simulink model "TestHeightController"  (R2020b)
settings: Solver=VariableStepAuto  StartTime=0.0  StopTime=10.0  RelTol=1e-3
undefined symbols (not defined in the file): Initial, Uav
libraries: pid_lib x1
settings Model: Creator=jban039  LastModifiedBy=jeremie
settings DebuggingCC: ArithmeticOperatorsInVariantConditions=warning
settings SFSimCC: SimUseLocalCustomCode=off  CustomCodeUndefinedFunction=UseInterfaceOnly
settings RTWCC: RTWUseLocalCustomCode=off

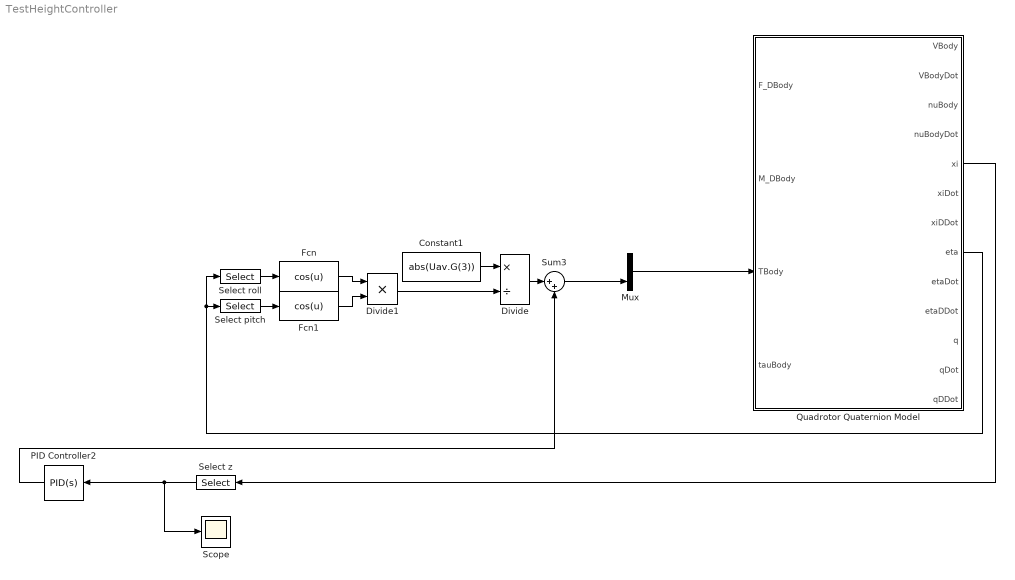
== system TestHeightController ==
  Constant1 : Constant  Value=abs(Uav.G(3))
  Divide : Product  Inputs=*/
  Divide1 : Product  Inputs=**
  Fcn : Fcn  Expr=cos(u)
  Fcn1 : Fcn  Expr=cos(u)
  Mux : Mux  Inputs=3
  PID Controller2 : pid_lib/PID Controller  Controller=PID  Form=Parallel  TimeDomain=Continuous-time  UseExternalTs=off  SampleTime=-1  IntegratorMethod=Forward Euler  FilterMethod=Forward Euler  ControllerParametersSource=internal  P=-22.065410118279  I=-10.2297340963903  D=-11.7817329577601  UseFilter=on  N=104.897155810233  TunerSelectOption=Transfer Function Based (PID Tuner App)  InitialConditionSource=internal  InitialConditionForIntegrator=0  InitialConditionForFilter=0  DifferentiatorICPrevScaledInput=0  ExternalReset=none  TrackingMode=off  Kt=1  LimitOutput=off  SatLimitsSource=internal  UpperSaturationLimit=inf  LowerSaturationLimit=-inf  LinearizeAsGain=on  AntiWindupMode=none  Kb=1  POutMin=[]  POutMax=[]  IOutMin=[]  IOutMax=[]  DOutMin=[]  DOutMax=[]  NOutMin=[]  NOutMax=[]  SumOutMin=[]  SumOutMax=[]  SaturationOutMin=[]  SaturationOutMax=[]  PParamMin=[]  PParamMax=[]  IParamMin=[]  IParamMax=[]  DParamMin=[]  DParamMax=[]  NParamMin=[]  NParamMax=[]  KbParamMin=[]  KbParamMax=[]  KtParamMin=[]  KtParamMax=[]  KbOutMin=[]  KbOutMax=[]  KtOutMin=[]  KtOutMax=[]  IntegratorOutMin=[]  IntegratorOutMax=[]  FilterOutMin=[]  FilterOutMax=[]  SumI1OutMin=[]  SumI1OutMax=[]  SumI2OutMin=[]  SumI2OutMax=[]  SumI3OutMin=[]  SumI3OutMax=[]  SumI4OutMin=[]  SumI4OutMax=[]  SumDOutMin=[]  SumDOutMax=[]  DifferentiatorOutMin=[]  DifferentiatorOutMax=[]  FilterDiffOutCoefMin=[]  FilterDiffOutCoefMax=[]  ReciprocalOutMin=[]  ReciprocalOutMax=[]  SumDenOutMin=[]  SumDenOutMax=[]  SumNumOutMin=[]  SumNumOutMax=[]  DivideOutMin=[]  DivideOutMax=[]  UdiffTsProdOutMin=[]  UdiffTsProdOutMax=[]  NTsProdOutMin=[]  NTsProdOutMax=[]  UintegralTsProdOutMin=[]  UintegralTsProdOutMax=[]  UngainTsProdOutMin=[]  UngainTsProdOutMax=[]  IntegratorContinuousStateAttributes=''  IntegratorStateMustResolveToSignalObject=off  IntegratorRTWStateStorageClass=Auto  FilterContinuousStateAttributes=''  FilterStateMustResolveToSignalObject=off  FilterRTWStateStorageClass=Auto  ParallelPVariant=InternalParameters  IdealPVariant=Disabled  IVariant=InternalParameters  DVariant=InternalParameters  IntegratorVariant=Continuous  SatVariant=Disabled  AWVariant=Passthrough  PCopyVariant=Disabled  TRVariant=Disabled  FdbkBlocksVariant=Forward  IdealPFdbkVariant=Disabled  SatFdbkVariant=Disabled  DerivativeFilterVariant=ContFilter  NVariant=InternalParameters  NCopyVariant=Disabled  FilterICVariant=InternalICsFilter  IntegratorICVariant=InternalICs  ExternalResetVariant=Disabled  TRSumVariant=Passthrough  SumFdbkVariant=Disabled  SumVariant=Sum_PID  TsampFilterVariant=InternalTs  TsampNgainVariant=Passthrough  TsampIntegralVariant=Passthrough  ExternalSaturationOutDataTypeStr=Inherit: Same as second input
  Quadrotor Quaternion Model : Subsystem
  Scope : Scope
  Select pitch : Selector  InputPortWidth=3  IndexOptions=Index vector (dialog)  Indices=2  OutputSizes=1
  Select roll : Selector  InputPortWidth=3  IndexOptions=Index vector (dialog)  Indices=1  OutputSizes=1
  Select z : Selector  InputPortWidth=3  IndexOptions=Index vector (dialog)  Indices=3  OutputSizes=1
  Sum3 : Sum  Inputs=|++
  wires:
  PID Controller2/1 -> Sum3/2
  Divide1/1 -> Divide/2
  Fcn1/1 -> Divide1/2
  Fcn/1 -> Divide1/1
  Select pitch/1 -> Fcn1/1
  Select roll/1 -> Fcn/1
  Quadrotor Quaternion Model/8(eta) -> Select pitch/1, Select roll/1
  Constant1/1 -> Divide/1
  Divide/1 -> Sum3/1
  Sum3/1 -> Mux/3
  Mux/1 -> Quadrotor Quaternion Model/3(TBody)
  Quadrotor Quaternion Model/5(xi) -> Select z/1
  Select z/1 -> Scope/1, PID Controller2/1

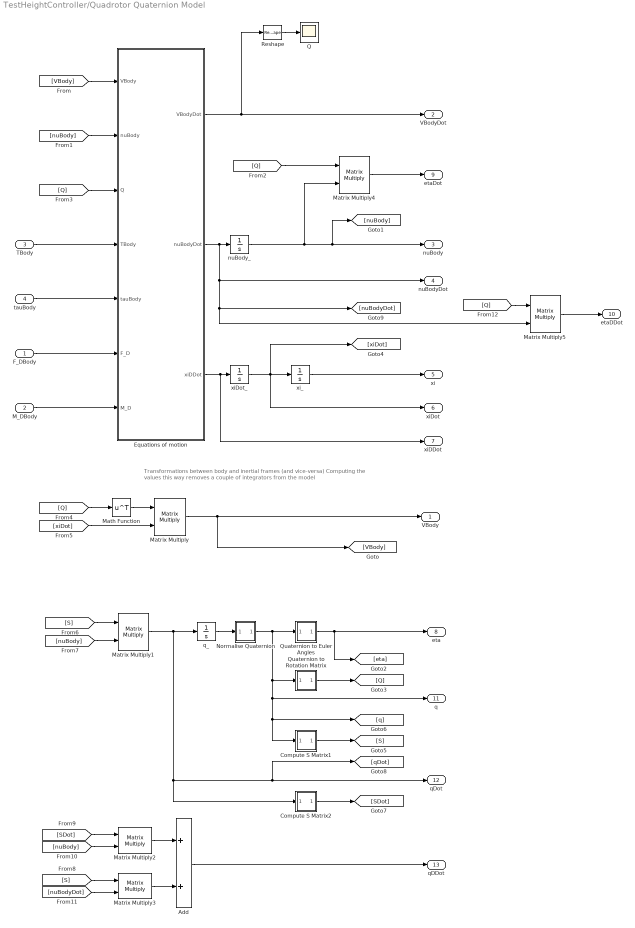
== system TestHeightController/Quadrotor Quaternion Model ==
  note: Transformations between body and inertial frames (and vice-versa)
      | Computing the values this way removes a couple of integrators from the model
  F_DBody : Inport  Unit=N
  M_DBody : Inport  Port=2  Unit=N*m
  TBody : Inport  Port=3  Unit=N
  tauBody : Inport  Port=4  Unit=N*m
  Add : Sum
  Compute S Matrix1 : Subsystem  AncestorBlock=QuaternionLibrary/Compute S Matrix
      mask help: Convert an orientation quaternion to an orthogonal transformation matrix
      mask Help:
      | Convert a quaternion
      | [q1 q2 q3 q4]
      | to the S matrix used to compute angular acceleration and velocity quaternion
      | qDot = S * nuBody
      | 
      | qDDot = SDot * nuBody + S * nuBodyDot
      mask Display: disp('S')
  Compute S Matrix2 : Subsystem  AncestorBlock=QuaternionLibrary/Compute S Matrix
      mask help: Convert an orientation quaternion to an orthogonal transformation matrix
      mask Help:
      | Convert a quaternion
      | [q1 q2 q3 q4]
      | to the S matrix used to compute angular acceleration and velocity quaternion
      | qDot = S * nuBody
      | 
      | qDDot = SDot * nuBody + S * nuBodyDot
      mask Display: disp('S')
  Equations of motion : MATLAB Function  TreatAsAtomicUnit=on
  Math Function : Math  Operator=transpose  SignedPower=on  SaturateOnIntegerOverflow=on
  Matrix Multiply{,1..5} (6 alike) : Product  Multiplication=Matrix(*)
  Normalise Quaternion : Subsystem  AncestorBlock=QuaternionLibrary/Normalise Quaternion
      mask help:
      | Normalise a quaternion
      |
      | Qhat = Q / |Q|
      mask Display: disp('Q/|Q|')
  Q : Scope
  Quaternion to Euler Angles : Subsystem  AncestorBlock=QuaternionLibrary/Quaternion to Euler Angles
      mask help: Convert an orientation quaternion to a vector of Euler angles
      mask Help:
      | Convert an orientation quaternion
      | [q1 q2 q3 q4]
      | where:
      | - q1 is the rotation in radians
      | - [q2 q3 q4] is the vector around which the rotation is performed)
      | to a vector of Euler angles
      | [roll, pitch, yaw]
      | Based on code from the PX4 firmware: https://github.com/PX4/Firmware
      mask Display: disp('Q2E')
  Quaternion to Rotation Matrix : Subsystem  AncestorBlock=QuaternionLibrary/Quaternion to Rotation Matrix
      mask help: Convert an orientation quaternion to an orthogonal transformation matrix
      mask Help:
      | Convert an orientation quaternion
      | [q1 q2 q3 q4]
      | where:
      | - q1 is the rotation in radians
      | - [q2 q3 q4] is the vector around which the rotation is performed)
      | to an orthogonal transformation matrix
      | Based on code from the PX4 firmware: https://github.com/PX4/Firmware
      mask Display: disp('Q2R')
  Reshape : Reshape  OutputDimensionality=Column vector (2-D)
  nuBody_ : Integrator  InitialCondition=Initial.NU_BODY
  q_ : Integrator  InitialCondition=Initial.Q
  xiDot_ : Integrator  InitialCondition=Initial.XI_DOT
  xi_ : Integrator  InitialCondition=[0;0;0.01]
  VBody : Outport  Unit=m/s  VectorParamsAs1DForOutWhenUnconnected=off
  VBodyDot : Outport  Port=2  Unit=m/s^2  VectorParamsAs1DForOutWhenUnconnected=off
  nuBody : Outport  Port=3  Unit=rad/s  VectorParamsAs1DForOutWhenUnconnected=off
  nuBodyDot : Outport  Port=4  Unit=rad/s^2  VectorParamsAs1DForOutWhenUnconnected=off
  xi : Outport  Port=5  Unit=m  VectorParamsAs1DForOutWhenUnconnected=off
  xiDot : Outport  Port=6  Unit=m/s  VectorParamsAs1DForOutWhenUnconnected=off
  xiDDot : Outport  Port=7  Unit=m/s^2  VectorParamsAs1DForOutWhenUnconnected=off
  eta : Outport  Port=8  Unit=rad  VectorParamsAs1DForOutWhenUnconnected=off
  etaDot : Outport  Port=9  Unit=rad/s  VectorParamsAs1DForOutWhenUnconnected=off
  etaDDot : Outport  Port=10  Unit=rad/s^2  VectorParamsAs1DForOutWhenUnconnected=off
  q : Outport  Port=11  VectorParamsAs1DForOutWhenUnconnected=off
  qDot : Outport  Port=12  VectorParamsAs1DForOutWhenUnconnected=off
  qDDot : Outport  Port=13  VectorParamsAs1DForOutWhenUnconnected=off
  wires:
  xiDot_/1 -> xiDot/1, [xiDot], xi_/1
  Reshape/1 -> Q/1
  Matrix Multiply5/1 -> etaDDot/1
  [Q] -> Matrix Multiply5/1
  Add/1 -> qDDot/1
  [Q] -> Matrix Multiply4/1
  Compute S Matrix1/1(rotationMatrix) -> [S]
  Normalise Quaternion/1(normalised) -> Quaternion to Rotation Matrix/1(quaternion), [q], Compute S Matrix1/1(quaternion), q/1, Quaternion to Euler Angles/1(quaternion)
  Matrix Multiply3/1 -> Add/2
  Matrix Multiply2/1 -> Add/1
  [nuBodyDot] -> Matrix Multiply3/2
  [nuBody] -> Matrix Multiply2/2
  [SDot] -> Matrix Multiply2/1
  Matrix Multiply1/1 -> q_/1, Compute S Matrix2/1(quaternion), [qDot], qDot/1
  [S] -> Matrix Multiply3/1
  Compute S Matrix2/1(rotationMatrix) -> [SDot]
  [nuBody] -> Matrix Multiply1/2
  [S] -> Matrix Multiply1/1
  Math Function/1 -> Matrix Multiply/1
  [xiDot] -> Matrix Multiply/2
  [Q] -> Math Function/1
  [Q] -> Equations of motion/3(Q)
  Quaternion to Rotation Matrix/1(rotationMatrix) -> [Q]
  Matrix Multiply4/1 -> etaDot/1
  Quaternion to Euler Angles/1(euler) -> [eta], eta/1
  q_/1 -> Normalise Quaternion/1(quaternion)
  Equations of motion/2(nuBodyDot) -> [nuBodyDot], Matrix Multiply5/2, nuBodyDot/1, nuBody_/1
  nuBody_/1 -> nuBody/1, [nuBody], Matrix Multiply4/2
  M_DBody/1 -> Equations of motion/7(M_D)
  Matrix Multiply/1 -> [VBody], VBody/1
  F_DBody/1 -> Equations of motion/6(F_D)
  Equations of motion/3(xiDDot) -> xiDDot/1, xiDot_/1
  TBody/1 -> Equations of motion/4(TBody)
  tauBody/1 -> Equations of motion/5(tauBody)
  [VBody] -> Equations of motion/1(VBody)
  [nuBody] -> Equations of motion/2(nuBody)
  xi_/1 -> xi/1
  Equations of motion/1(VBodyDot) -> VBodyDot/1, Reshape/1

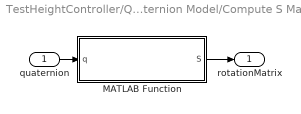
== system TestHeightController/Quadrotor Quaternion Model/Compute S Matrix1 ==
  quaternion : Inport
  MATLAB Function : MATLAB Function  TreatAsAtomicUnit=on
  rotationMatrix : Outport  VectorParamsAs1DForOutWhenUnconnected=off
  wires:
  quaternion/1 -> MATLAB Function/1(q)
  MATLAB Function/1(S) -> rotationMatrix/1

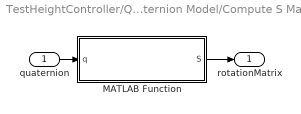
== system TestHeightController/Quadrotor Quaternion Model/Compute S Matrix2 ==
  quaternion : Inport
  MATLAB Function : MATLAB Function  TreatAsAtomicUnit=on
  rotationMatrix : Outport  VectorParamsAs1DForOutWhenUnconnected=off
  wires:
  quaternion/1 -> MATLAB Function/1(q)
  MATLAB Function/1(S) -> rotationMatrix/1

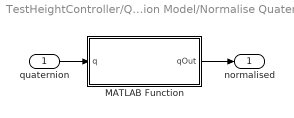
== system TestHeightController/Quadrotor Quaternion Model/Normalise Quaternion ==
  quaternion : Inport
  MATLAB Function : MATLAB Function  TreatAsAtomicUnit=on
  normalised : Outport  VectorParamsAs1DForOutWhenUnconnected=off
  wires:
  quaternion/1 -> MATLAB Function/1(q)
  MATLAB Function/1(qOut) -> normalised/1

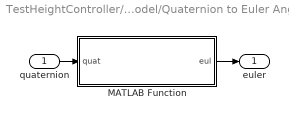
== system TestHeightController/Quadrotor Quaternion Model/Quaternion to Euler Angles ==
  quaternion : Inport
  MATLAB Function : MATLAB Function  TreatAsAtomicUnit=on
  euler : Outport  VectorParamsAs1DForOutWhenUnconnected=off
  wires:
  quaternion/1 -> MATLAB Function/1(quat)
  MATLAB Function/1(eul) -> euler/1

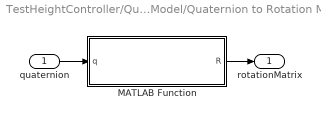
== system TestHeightController/Quadrotor Quaternion Model/Quaternion to Rotation Matrix ==
  quaternion : Inport
  MATLAB Function : MATLAB Function  TreatAsAtomicUnit=on
  rotationMatrix : Outport  VectorParamsAs1DForOutWhenUnconnected=off
  wires:
  MATLAB Function/1(R) -> rotationMatrix/1
  quaternion/1 -> MATLAB Function/1(q)

== matlab function TestHeightController/Quadrotor Quaternion Model/Equations of motion ==
  data: VBody input; VBodyDot output; nuBody input; Q input; TBody input size=3; tauBody input size=3; F_D input size=3; M_D input size=3; nuBodyDot output; Uav parameter; xiDDot output
function [VBodyDot, nuBodyDot, xiDDot] = QuadrotorQuaternionModel(...
    VBody, nuBody, Q, TBody, tauBody, F_D, M_D, Uav)
%#codegen

%% Rotation matrices

%% Moments and Forces
% Body frame accelerations
VBodyDot  = (1/Uav.M) * (Q'*Uav.G + TBody - cross(nuBody, Uav.M*VBody) - F_D);
nuBodyDot = Uav.I \ (tauBody - cross(nuBody, Uav.I*nuBody) - M_D);

% Inertial frame accelerations
xiDDot = (1/Uav.M)*(Uav.G + Q*(TBody - F_D));
% etaDDot = WInvertDot*nuBody + WInvert*nuBodyDot;

% Check centripetal force in inertial frame
% F_C = R*cross(nuBody,m*VBody);
end

== matlab function TestHeightController/Quadrotor Quaternion Model/Quaternion to Rotation Matrix/MATLAB Function ==
  data: q input; R output
function R = QuatToRot( q )
%QUATTOROT Convert quaternion to rotation matrix
%   Written by:    J.X.J. Bannwarth, 2017/03/27
%   Last modified: J.X.J. Bannwarth, 2018/12/11
    W = q(1);
    X = q(2);
    Y = q(3);
    Z = q(4);
    
    xx = X * X;
    xy = X * Y;
    xz = X * Z;
    xw = X * W;

    yy = Y * Y;
    yz = Y * Z;
    yw = Y * W;
    
    zz = Z * Z;
    zw = Z * W;

    m00 = 1 - 2 * ( yy + zz );
    m01 =     2 * ( xy - zw );
    m02 =     2 * ( xz + yw );

    m10 =     2 * ( xy + zw );
    m11 = 1 - 2 * ( xx + zz );
    m12 =     2 * ( yz - xw );

    m20 =     2 * ( xz - yw );
    m21 =     2 * ( yz + xw );
    m22 = 1 - 2 * ( xx + yy );
    
    R = [m00 m01 m02;
         m10 m11 m12;
         m20 m21 m22];   
end

== matlab function TestHeightController/Quadrotor Quaternion Model/Quaternion to Euler Angles/MATLAB Function ==
  data: quat input; eul output
function eul   = QuaternionToEuler( quat )
%QUATERNIONTOEULER Convert quaternion to euler angles
%   Based on PX4 Firmware code: https://github.com/PX4/Firmware
%   Written by:    J.X.J. Bannwarth, 2016/08/29
%   Last modified: J.X.J. Bannwarth, 2018/12/11

    eul = [ atan2(2.0 .* (quat(1) .* quat(2) + quat(3) .* quat(4)), ...
                1.0 - 2.0 .* (quat(2) .* quat(2) + quat(3) .* quat(3)));
	        asin(2.0 .* (quat(1) .* quat(3) - quat(4) .* quat(2)));
            atan2(2.0 .* (quat(1) .* quat(4) + quat(2) .* quat(3)), ...
                1.0 - 2.0 .* (quat(3) .* quat(3) + quat(4) .* quat(4))) ];
end

== matlab function TestHeightController/Quadrotor Quaternion Model/Compute S Matrix2/MATLAB Function ==
  data: q input; S output
function S = ComputeSMatrix(q)
%COMPUTESMATRIX Compute S Matrix
%   Written by:    J.X.J. Bannwarth, 2017/03/28
%   Last modified: J.X.J. Bannwarth, 2018/12/11
    S = zeros( 4, 3 );
    S(1,1) = -q(2) * 0.5;
    S(1,2) = -q(3) * 0.5;
    S(1,3) = -q(4) * 0.5;
    S(2,1) =  q(1) * 0.5;
    S(2,2) = -q(4) * 0.5;
    S(2,3) =  q(3) * 0.5;
    S(3,1) =  q(4) * 0.5;
    S(3,2) =  q(1) * 0.5;
    S(3,3) = -q(2) * 0.5;
    S(4,1) = -q(3) * 0.5;
    S(4,2) =  q(2) * 0.5;
    S(4,3) =  q(1) * 0.5;
end

== matlab function TestHeightController/Quadrotor Quaternion Model/Normalise Quaternion/MATLAB Function ==
  data: q input; qOut output
function qOut = NormaliseQuat( q )
%NORMALISEQUAT Normalise quaternion
%   Based on PX4 Firmware code: https://github.com/PX4/Firmware
%   Written by:    J.X.J. Bannwarth, 2018/12/11
%   Last modified: J.X.J. Bannwarth, 2018/12/11

    qOut = zeros(4,1);
    normVal = sqrt( dot( q, q ) );
    if normVal ~= 0
        qOut = q ./ normVal;
    end
end

== matlab function TestHeightController/Quadrotor Quaternion Model/Compute S Matrix1/MATLAB Function ==
  data: q input; S output
function S = ComputeSMatrix(q)
%COMPUTESMATRIX Compute S Matrix
%   Written by:    J.X.J. Bannwarth, 2017/03/28
%   Last modified: J.X.J. Bannwarth, 2018/12/11
    S = zeros( 4, 3 );
    S(1,1) = -q(2) * 0.5;
    S(1,2) = -q(3) * 0.5;
    S(1,3) = -q(4) * 0.5;
    S(2,1) =  q(1) * 0.5;
    S(2,2) = -q(4) * 0.5;
    S(2,3) =  q(3) * 0.5;
    S(3,1) =  q(4) * 0.5;
    S(3,2) =  q(1) * 0.5;
    S(3,3) = -q(2) * 0.5;
    S(4,1) = -q(3) * 0.5;
    S(4,2) =  q(2) * 0.5;
    S(4,3) =  q(1) * 0.5;
end
